simulink model "FIN_CARRERA_IZAJE"  (R2023a)
settings: Solver=VariableStepAuto  StartTime=0.0  StopTime=10.0  RelTol=1e-3
undefined symbols (not defined in the file): Yt0
settings Model: Creator=Ignacio  LastModifiedBy=Ignacio

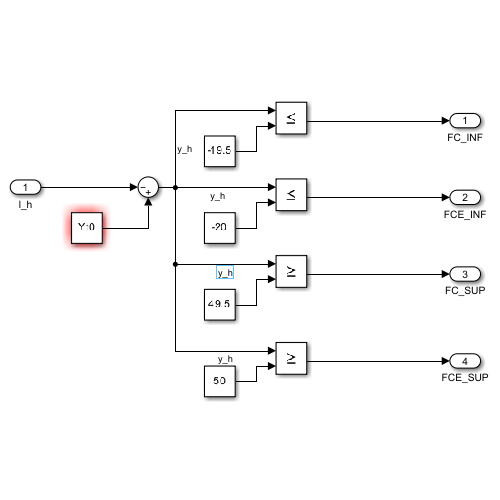
[thumbnail: Simulink's stored preview of the top-level diagram]
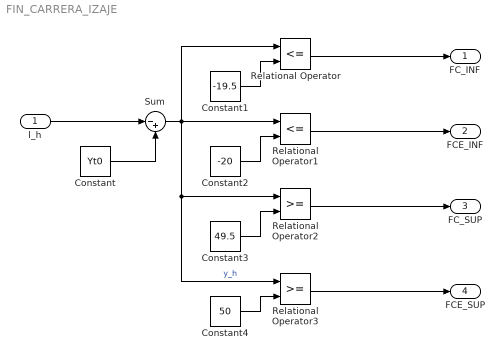
== system FIN_CARRERA_IZAJE ==
  l_h : Inport
  Constant : Constant  Value=Yt0
  Constant1 : Constant  Value=-19.5
  Constant2 : Constant  Value=-20
  Constant3 : Constant  Value=49.5
  Constant4 : Constant  Value=50
  Relational Operator : RelationalOperator  Operator=<=  OutDataTypeStr=boolean  RndMeth=Simplest  InputSameDT=off
  Relational Operator1 : RelationalOperator  Operator=<=  OutDataTypeStr=boolean  RndMeth=Simplest  InputSameDT=off
  Relational Operator2 : RelationalOperator  OutDataTypeStr=boolean  RndMeth=Simplest  InputSameDT=off
  Relational Operator3 : RelationalOperator  OutDataTypeStr=boolean  RndMeth=Simplest  InputSameDT=off
  Sum : Sum  Inputs=|-+
  FC_INF : Outport
  FCE_INF : Outport  Port=2
  FC_SUP : Outport  Port=3
  FCE_SUP : Outport  Port=4
  wires:
  l_h/1 -> Sum/1
  Constant/1 -> Sum/2
  Relational Operator/1 -> FC_INF/1
  Constant1/1 -> Relational Operator/2
  Constant2/1 -> Relational Operator1/2
  Relational Operator1/1 -> FCE_INF/1
  Constant3/1 -> Relational Operator2/2
  Relational Operator2/1 -> FC_SUP/1
  Relational Operator3/1 -> FCE_SUP/1
  Constant4/1 -> Relational Operator3/2
  Sum/1 -> Relational Operator3/1, Relational Operator2/1, Relational Operator/1, Relational Operator1/1  "y_h"
